simulink model "E2_3"  (R2022a)
settings: Solver=VariableStepAuto  StartTime=0.0  StopTime=50  MaxStep=0.001  RelTol=1e-3
InitFcn:
  | sigma=10;
  | rho=28;
  | beta=8/3;
  | X0=1;
  | Y0=1;
  | Z0=1;
settings Model: Creator=Reza  LastModifiedBy=Reza

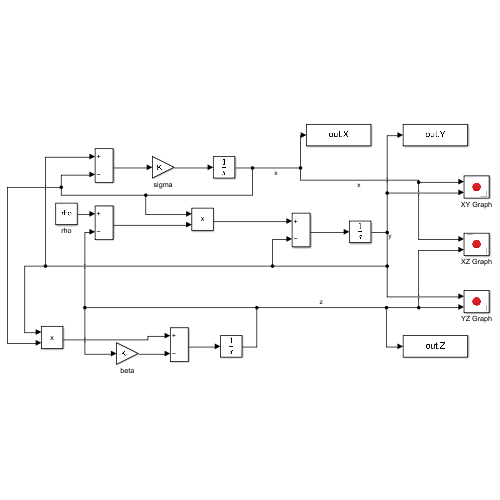
[thumbnail: Simulink's stored preview of the top-level diagram]
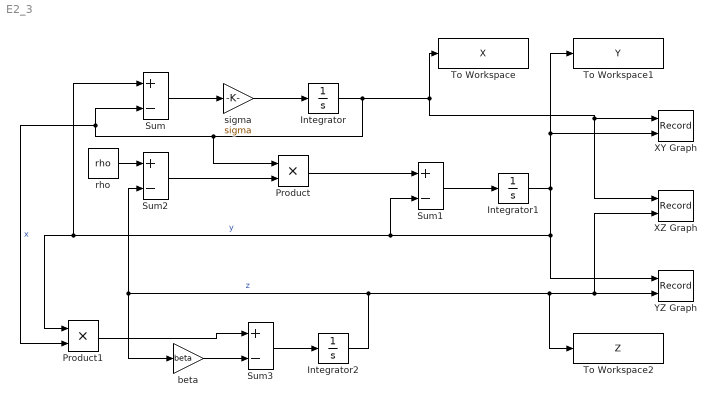
== system E2_3 ==
  Integrator : Integrator  InitialCondition=X0
  Integrator1 : Integrator  InitialCondition=Y0
  Integrator2 : Integrator  InitialCondition=Z0
  Product : Product
  Product1 : Product
  Sum{,1..3} (4 alike) : Sum  Inputs=+-
  To Workspace : ToWorkspace  VariableName=X  SampleTime=-1
  To Workspace1 : ToWorkspace  VariableName=Y  SampleTime=-1
  To Workspace2 : ToWorkspace  VariableName=Z  SampleTime=-1
  XY Graph : Record  FileSettingsInternal="{\"entries\":[{\"content\":{\"excelSettings\":{\"content\":{},\"type\":\"Streamout.ExcelSettings\"}},\"type\":\"Streamout.FileSettingStorage\",\"uuid\":\"d5e8e67d-65f5-439d-baf3-5cfe0ea3069c\"}],\"packageUris\":[\"http://schema.mathworks.com/mf0/streamout_blocks/R2020a\"],\"version\":\"1.0\"}"  Layout=[1 1]  SignalsInternal="{\"entries\":[{\"content\":{\"signals\":[{\"content\":{\"blockPath\":[\"E2_3/XY Graph\"],\"channel\":[],\"dimensions\":[1],\"domain\":\"E2_3/XY Graph\",\"lineColor\":\"#edb120\",\"plots\":[],\"port\":1,\"sid\":[\"\"],\"signalID\":341,\"signalName\":\"x\"},\"type\":\"RecordBlkView.Signal\",\"uuid\":\"27801372-b7ba-455c-83ab-0dae9fb10c2f\"},{\"content\":{\"blockPath\":[\"E2_3/XY Graph\"],\"channel\":[],\"dimensions\":[1],\"domain\":\"E2_3/XY Graph\",\"lineColor\":\"#7e2f8e\",\"plots\":[],\"port\":2,\"sid\":[\"\"],\"signalID\":345,\"signalName\":\"y\"},\"type\":\"RecordBlkView.Signal\",\"uuid\":\"7f056ca5-6b0a-4d6c-b88e-bd8a10d10ed1\"}]},\"type\":\"RecordBlkView.InputSignals\",\"uuid\":\"93b13b71-ce58-4ec2-a4aa-9f660e82d8ca\"}],\"packageUris\":[\"http://schema.mathworks.com/mf0/streamout_blocks/R2020a\"],\"version\":\"1.0\"}"  VisualizationBindings="{\"xyplotplugin\":{\"info\":[{\"series\":[],\"subplotID\":1}]}}"  CompatibilityTag=XY
  XZ Graph : Record  FileSettingsInternal="{\"entries\":[{\"content\":{\"excelSettings\":{\"content\":{},\"type\":\"Streamout.ExcelSettings\"}},\"type\":\"Streamout.FileSettingStorage\",\"uuid\":\"8417785a-8a9f-43dc-9b60-5e8633ed2ac2\"}],\"packageUris\":[\"http://schema.mathworks.com/mf0/streamout_blocks/R2020a\"],\"version\":\"1.0\"}"  Layout=[1 1]  SignalsInternal="{\"entries\":[{\"content\":{\"signals\":[{\"content\":{\"blockPath\":[\"E2_3/XZ Graph\"],\"channel\":[],\"dimensions\":[1],\"domain\":\"E2_3/XZ Graph\",\"lineColor\":\"#77ac30\",\"plots\":[],\"port\":1,\"sid\":[\"\"],\"signalID\":349,\"signalName\":\"x\"},\"type\":\"RecordBlkView.Signal\",\"uuid\":\"21979492-c1fc-4b5b-8984-de8e808e6029\"},{\"content\":{\"blockPath\":[\"E2_3/XZ Graph\"],\"channel\":[],\"dimensions\":[1],\"domain\":\"E2_3/XZ Graph\",\"lineColor\":\"#4dbeee\",\"plots\":[],\"port\":2,\"sid\":[\"\"],\"signalID\":353,\"signalName\":\"z\"},\"type\":\"RecordBlkView.Signal\",\"uuid\":\"4338ce35-d9c4-400a-9c35-3bbdb2ca0530\"}]},\"type\":\"RecordBlkView.InputSignals\",\"uuid\":\"3fd1bed5-9066-4c97-957c-7891df3cf5bf\"}],\"packageUris\":[\"http://schema.mathworks.com/mf0/streamout_blocks/R2020a\"],\"version\":\"1.0\"}"  VisualizationBindings="{\"xyplotplugin\":{\"info\":[{\"series\":[],\"subplotID\":1}]}}"  CompatibilityTag=XY
  YZ Graph : Record  FileSettingsInternal="{\"entries\":[{\"content\":{\"excelSettings\":{\"content\":{},\"type\":\"Streamout.ExcelSettings\"}},\"type\":\"Streamout.FileSettingStorage\",\"uuid\":\"93e8490c-106e-4821-a1e8-deccf6a70005\"}],\"packageUris\":[\"http://schema.mathworks.com/mf0/streamout_blocks/R2020a\"],\"version\":\"1.0\"}"  Layout=[1 1]  SignalsInternal="{\"entries\":[{\"content\":{\"signals\":[{\"content\":{\"blockPath\":[\"E2_3/YZ Graph\"],\"channel\":[],\"dimensions\":[1],\"domain\":\"E2_3/YZ Graph\",\"lineColor\":\"#a2142f\",\"plots\":[],\"port\":1,\"sid\":[\"\"],\"signalID\":357,\"signalName\":\"y\"},\"type\":\"RecordBlkView.Signal\",\"uuid\":\"31b0451c-853f-492d-9b4a-180c6c12fc6f\"},{\"content\":{\"blockPath\":[\"E2_3/YZ Graph\"],\"channel\":[],\"dimensions\":[1],\"domain\":\"E2_3/YZ Graph\",\"lineColor\":\"#139fff\",\"plots\":[],\"port\":2,\"sid\":[\"\"],\"signalID\":361,\"signalName\":\"z\"},\"type\":\"RecordBlkView.Signal\",\"uuid\":\"53dabc59-9f7b-49cb-a35d-4da9fb9d58a9\"}]},\"type\":\"RecordBlkView.InputSignals\",\"uuid\":\"5de9ced1-384f-4995-9ef9-9e16af4a04fe\"}],\"packageUris\":[\"http://schema.mathworks.com/mf0/streamout_blocks/R2020a\"],\"version\":\"1.0\"}"  VisualizationBindings="{\"xyplotplugin\":{\"info\":[{\"series\":[],\"subplotID\":1}]}}"  CompatibilityTag=XY
  beta : Gain  Gain=beta
  rho : Constant  Value=rho
  sigma : Gain  Gain=sigma
  wires:
  sigma/1 -> Integrator/1
  Sum/1 -> sigma/1
  Integrator1/1 -> XY Graph/2, To Workspace1/1, YZ Graph/1, Sum1/2, Product1/1, Sum/1  "y"
  Integrator/1 -> XZ Graph/1, XY Graph/1, To Workspace/1, Product/1, Product1/2, Sum/2  "x"
  rho/1 -> Sum2/1
  Integrator2/1 -> XZ Graph/2, YZ Graph/2, To Workspace2/1, beta/1, Sum2/2  "z"
  Sum2/1 -> Product/2
  Product/1 -> Sum1/1
  Sum1/1 -> Integrator1/1
  Sum3/1 -> Integrator2/1
  beta/1 -> Sum3/2
  Product1/1 -> Sum3/1
